simulink model "sim_system_lin"  (Simulink 7.9)
settings: Solver=ode45  StartTime=0.0  StopTime=30  RelTol=1e-3
values from neighbouring files (symbols this model uses):
  A_lin = J    [linearisation.m]
  B_lin = [B_lin_Wf B_lin_Ccharge]    [linearisation.m]
  C_charge_0 = f_ctl(Wf_0, Ng_0)    [point_equilibre.m]
  C_lin = [0 1 0 ... (first row only)    [linearisation.m]
  D_lin = [0 0 ... (first row only)    [linearisation.m]
  Ng_0 = 28000    [point_equilibre.m]
  Ntl_0 = ntlnom    [point_equilibre.m]
  ss_capteur_temperature = ss(A_capteur_temperature, B_capteur_temperature, C_capteur_temperature, D_capteur_temperature)    [ss_doseur_capteur.m]
  ss_doseur = ss(tf([1],[tdos 1]))    [ss_doseur_capteur.m]
  T45_0 = f_t45(Wf_0, Ng_0)    [point_equilibre.m]
  Wf_0 = fminsearch(@(wf) abs(f_cg(wf,28000)), Wf_init)    [point_equilibre.m]
settings Model: Creator=maffre  LastModifiedBy=maffre

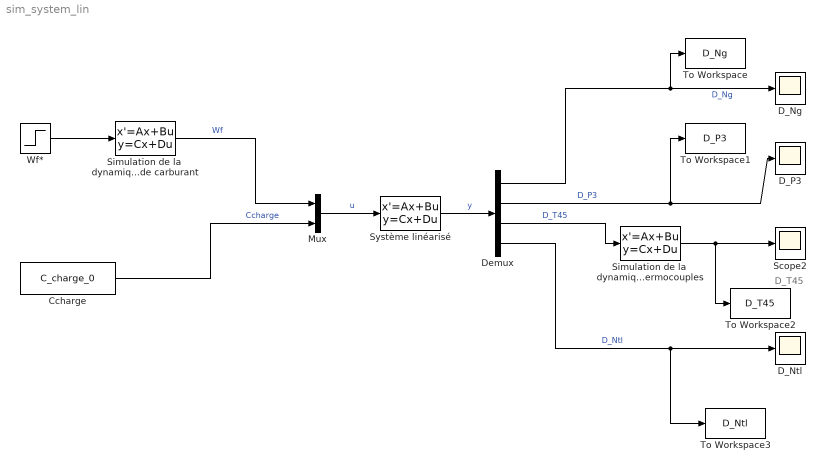
== system sim_system_lin ==
  note: D_T45
  Ccharge : Constant  Value=C_charge_0
  D_Ng : Scope
  D_Ntl : Scope
      settings: SaveName=ScopeData3
  D_P3 : Scope
  Demux : Demux
  Mux : Mux  Inputs=2
  Scope2 : Scope
      settings: SaveName=ScopeData2
  Simulation de la  dynamique des  thermocouples : StateSpace  A=ss_capteur_temperature.A  B=ss_capteur_temperature.B  C=ss_capteur_temperature.C  D=ss_capteur_temperature.D  X0=T45_0
  Simulation de la  dynamique du doseur  de carburant : StateSpace  A=ss_doseur.A  B=ss_doseur.B  C=ss_doseur.C  D=ss_doseur.D  X0=Wf_0
  Système linéarisé : StateSpace  A=A_lin  B=B_lin  C=C_lin  D=D_lin  X0=[Wf_0 Ng_0 Ntl_0]
  To Workspace : ToWorkspace  VariableName=D_Ng  SampleTime=-1  SaveFormat=Timeseries
  To Workspace1 : ToWorkspace  VariableName=D_P3  SampleTime=-1  SaveFormat=Timeseries
  To Workspace2 : ToWorkspace  VariableName=D_T45  SampleTime=-1  SaveFormat=Timeseries
  To Workspace3 : ToWorkspace  VariableName=D_Ntl  SampleTime=-1  SaveFormat=Timeseries
  Wf* : Step  Time=10  Before=Wf_0  After=Wf_0 + 40  SampleTime=0
  wires:
  Système linéarisé/1 -> Demux/1  "y"
  Demux/1 -> D_Ng/1, To Workspace/1  "D_Ng"
  Demux/2 -> D_P3/1, To Workspace1/1  "D_P3"
  Demux/4 -> D_Ntl/1, To Workspace3/1  "D_Ntl"
  Mux/1 -> Système linéarisé/1  "u"
  Wf*/1 -> Simulation de la  dynamique du doseur  de carburant/1
  Simulation de la  dynamique du doseur  de carburant/1 -> Mux/1  "Wf"
  Ccharge/1 -> Mux/2  "Ccharge"
  Simulation de la  dynamique des  thermocouples/1 -> Scope2/1, To Workspace2/1
  Demux/3 -> Simulation de la  dynamique des  thermocouples/1  "D_T45"
